simulink model "simscape_actuation_22_withmotor"  (R2021a)
settings: Solver=VariableStepAuto  StartTime=0.001  StopTime=10  FixedStep=0.01  MaxStep=0.0001  RelTol=1e-4  AbsTol=1e-4
values from neighbouring files (symbols this model uses):
  As = 0.00025    [variables_5.mat]
  ext = 48232.2966308    [variables_5.mat]
  n = 0.912908754682    [variables_5.mat]
  ri = 0.00045    [variables_5.mat]
  ro = 0.0015    [variables_5.mat]
  Y = 7920.45919172    [variables_5.mat]
  yieldstress = 40000000    [variables_5.mat]
libraries: fl_lib x48, nesl_utility x17, fl_ps_legacy_lib x16, sh_lib x11, ee_lib x4, simulink x3, sdl_lib x2
(part 2 of 2)

== system simscape_actuation_22_withmotor/Controller (GIven by matlab)1/Position/Algorithm and Pulse Generation/IC Analog Output REV ==
  SL : Inport
  Controlled Voltage Source : fl_lib/Electrical/Electrical Sources/Controlled Voltage Source
      settings: SourceProductName=Foundation Library
  ERef : fl_lib/Electrical/Electrical Elements/Electrical Reference
      settings: SourceProductName=Foundation Library
  Simulink-PS Converter : nesl_utility/Simulink-PS Converter  PhysicalDomain=network_engine_domain  SubClassName=ps_input  LeftPortType=input  RightPortType=output  PseudoPeriodic=off  Frequencies=[]  NoiseDistribution=none  NoiseParameters=[]  Unit=V  AffineConversion=off  FilteringAndDerivatives=zero  SimscapeFilterOrder=1  InputFilterTimeConstant=.001  UdotUserProvided=0
      settings: SourceProductName=Utilities
  V : PMIOPort  Side=Right
  wires:
  SL/1 -> Simulink-PS Converter/1
  connections:
  Simulink-PS Converter/RConn1 -- Controlled Voltage Source/RConn1
  V/RConn1 -- Controlled Voltage Source/LConn1
  ERef/LConn1 -- Controlled Voltage Source/RConn2

== system simscape_actuation_22_withmotor/Controller (GIven by matlab)1/Position/Algorithm and Pulse Generation/IC Analog Output Vref ==
  SL : Inport
  Controlled Voltage Source : fl_lib/Electrical/Electrical Sources/Controlled Voltage Source
      settings: SourceProductName=Foundation Library
  ERef : fl_lib/Electrical/Electrical Elements/Electrical Reference
      settings: SourceProductName=Foundation Library
  Simulink-PS Converter : nesl_utility/Simulink-PS Converter  PhysicalDomain=network_engine_domain  SubClassName=ps_input  LeftPortType=input  RightPortType=output  PseudoPeriodic=off  Frequencies=[]  NoiseDistribution=none  NoiseParameters=[]  Unit=V  AffineConversion=off  FilteringAndDerivatives=zero  SimscapeFilterOrder=1  InputFilterTimeConstant=.001  UdotUserProvided=0
      settings: SourceProductName=Utilities
  V : PMIOPort  Side=Right
  wires:
  SL/1 -> Simulink-PS Converter/1
  connections:
  ERef/LConn1 -- Controlled Voltage Source/RConn2
  V/RConn1 -- Controlled Voltage Source/LConn1
  Simulink-PS Converter/RConn1 -- Controlled Voltage Source/RConn1

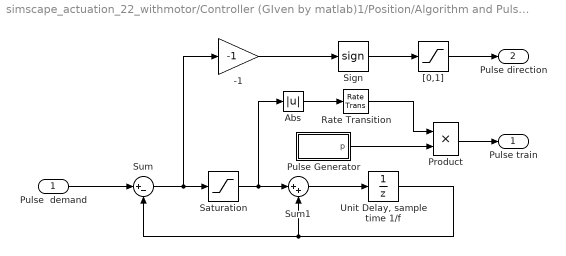
== system simscape_actuation_22_withmotor/Controller (GIven by matlab)1/Position/Algorithm and Pulse Generation/Pulse Generator ==
  Pulse  demand : Inport  SampleTime=1/f
  -1 : Gain  Gain=-1
  Abs : Abs
  Product : Product  InputSameDT=on  SaturateOnIntegerOverflow=on  OutDataTypeStr=Inherit: Same as first input
  Pulse Generator : Subsystem
  Rate Transition : RateTransition  Deterministic=off
  Saturation : Saturate  UpperLimit=1  LowerLimit=-1
  Sign : Signum
  Sum : Sum  Inputs=|+-
  Sum1 : Sum  Inputs=|++
  "Unit Delay, sample time 1/f" : UnitDelay  SampleTime=1/f  HasFrameUpgradeWarning=on
  "[0,1]" : Saturate  UpperLimit=1  LowerLimit=0
  Pulse train : Outport  VectorParamsAs1DForOutWhenUnconnected=off
  Pulse direction : Outport  Port=2  VectorParamsAs1DForOutWhenUnconnected=off
  wires:
  Rate Transition/1 -> Product/1
  Pulse Generator/1(p) -> Product/2
  Abs/1 -> Rate Transition/1
  Product/1 -> Pulse train/1
  Sign/1 -> "[0,1]"/1
  Sum1/1 -> "Unit Delay, sample time 1/f"/1
  Saturation/1 -> Abs/1, Sum1/1
  Sum/1 -> Saturation/1, -1/1
  Pulse  demand/1 -> Sum/1
  "Unit Delay, sample time 1/f"/1 -> Sum1/2, Sum/2
  -1/1 -> Sign/1
  "[0,1]"/1 -> Pulse direction/1

== system simscape_actuation_22_withmotor/Controller (GIven by matlab)1/Speed/Step Rate and Direction/IC Analog Output REV ==
  SL : Inport
  Controlled Voltage Source : fl_lib/Electrical/Electrical Sources/Controlled Voltage Source
      settings: SourceProductName=Foundation Library
  ERef : fl_lib/Electrical/Electrical Elements/Electrical Reference
      settings: SourceProductName=Foundation Library
  Simulink-PS Converter : nesl_utility/Simulink-PS Converter  PhysicalDomain=network_engine_domain  SubClassName=ps_input  LeftPortType=input  RightPortType=output  PseudoPeriodic=off  Frequencies=[]  NoiseDistribution=none  NoiseParameters=[]  Unit=V  AffineConversion=off  FilteringAndDerivatives=zero  SimscapeFilterOrder=1  InputFilterTimeConstant=.001  UdotUserProvided=0
      settings: SourceProductName=Utilities
  V : PMIOPort  Side=Right
  wires:
  SL/1 -> Simulink-PS Converter/1
  connections:
  ERef/LConn1 -- Controlled Voltage Source/RConn2
  V/RConn1 -- Controlled Voltage Source/LConn1
  Simulink-PS Converter/RConn1 -- Controlled Voltage Source/RConn1

== system simscape_actuation_22_withmotor/Controller (GIven by matlab)1/Speed/Step Rate and Direction/IC Analog Output Vref ==
  SL : Inport
  Controlled Voltage Source : fl_lib/Electrical/Electrical Sources/Controlled Voltage Source
      settings: SourceProductName=Foundation Library
  ERef : fl_lib/Electrical/Electrical Elements/Electrical Reference
      settings: SourceProductName=Foundation Library
  Simulink-PS Converter : nesl_utility/Simulink-PS Converter  PhysicalDomain=network_engine_domain  SubClassName=ps_input  LeftPortType=input  RightPortType=output  PseudoPeriodic=off  Frequencies=[]  NoiseDistribution=none  NoiseParameters=[]  Unit=V  AffineConversion=off  FilteringAndDerivatives=zero  SimscapeFilterOrder=1  InputFilterTimeConstant=.001  UdotUserProvided=0
      settings: SourceProductName=Utilities
  V : PMIOPort  Side=Right
  wires:
  SL/1 -> Simulink-PS Converter/1
  connections:
  Simulink-PS Converter/RConn1 -- Controlled Voltage Source/RConn1
  V/RConn1 -- Controlled Voltage Source/LConn1
  ERef/LConn1 -- Controlled Voltage Source/RConn2

== system simscape_actuation_22_withmotor/Controller (GIven by matlab)/Position/Algorithm and Pulse Generation/Pulse Generator/Pulse Generator ==
  -1 : Gain  Gain=0.5
  Constant : Constant  SampleTime=1/(2*f)
  Gain : Gain  Gain=-1
  Sum : Sum  Inputs=|++
  "Unit Delay, sample time 1/2*f)" : UnitDelay  InitialCondition=-1  SampleTime=1/(2*f)  HasFrameUpgradeWarning=on
  p : Outport  VectorParamsAs1DForOutWhenUnconnected=off
  wires:
  "Unit Delay, sample time 1/2*f)"/1 -> Gain/1, Sum/1
  Gain/1 -> "Unit Delay, sample time 1/2*f)"/1
  Constant/1 -> Sum/2
  Sum/1 -> -1/1
  -1/1 -> p/1

== system simscape_actuation_22_withmotor/Controller (GIven by matlab)1/Position/Algorithm and Pulse Generation/Pulse Generator/Pulse Generator ==
  -1 : Gain  Gain=0.5
  Constant : Constant  SampleTime=1/(2*f)
  Gain : Gain  Gain=-1
  Sum : Sum  Inputs=|++
  "Unit Delay, sample time 1/2*f)" : UnitDelay  InitialCondition=-1  SampleTime=1/(2*f)  HasFrameUpgradeWarning=on
  p : Outport  VectorParamsAs1DForOutWhenUnconnected=off
  wires:
  -1/1 -> p/1
  Sum/1 -> -1/1
  Constant/1 -> Sum/2
  Gain/1 -> "Unit Delay, sample time 1/2*f)"/1
  "Unit Delay, sample time 1/2*f)"/1 -> Sum/1, Gain/1
